simulink model "Fuzzy_Extended_State_Observer_Pendulum"  (R2019a)
settings: Solver=ode1  StartTime=0.0  StopTime=5  FixedStep=0.001  RelTol=1e-3
InitFcn:
  | %Variable_Entrada
  | Phi_max = 200;
  | Phi_2  = 10;
  | Phi_1  = 0.4;
  | Phi_0  = 0;
  | 
  | 
  | %Variable_Salida
  | U_2= 1;
  | U_1 =0.6;
  | U_0  = 0;
  | 
  | 
  | 
  | Phi_max2 = 200;
  | Phi_22  = 10;
  | Phi_12 = 0.3;
  | Phi_02  = 0;
  | 
  | U_22= 1;
  | U_12 =0.7;
  | U_02  = 0;
undefined symbols (not defined in the file or in its folder): fv, g, K, L, l, m
libraries: fuzblock x10, simulink x2
settings Model: Creator=DIEE  LastModifiedBy=dell
settings SolverCC: ZeroCrossAlgorithm=Adaptive
settings DataIOCC: LimitDataPoints=on  SaveFormat=Array  ReturnWorkspaceOutputs=off
settings OptimizationCC: BlockReduction=off  BooleanDataType=off  LifeSpan=inf
settings DebuggingCC: SaveWithParameterizedLinksMsg=none  UnderspecifiedInitializationDetection=Classic  MergeDetectMultiDrivingBlocksExec=none  SignalResolutionControl=TryResolveAllWithWarning  IgnoredZcDiagnostic=none  SFUnexpectedBacktrackingDiag=warning  SFNoUnconditionalDefaultTransitionDiag=warning  SFExecutionAtInitializationDiag=none  ArithmeticOperatorsInVariantConditions=warning
settings HardwareCC: ProdBitPerPointer=32  ProdBitPerSizeT=32  ProdBitPerPtrDiffT=32  ProdLargestAtomicFloat=None  ProdIntDivRoundTo=Undefined  ProdEndianess=Unspecified  ProdWordSize=32  ProdHWDeviceType=32-bit Generic  TargetUnknown=on
settings ModelReferenceCC: PropagateSignalLabelsOutOfModel=off
settings SFSimCC: SimUseLocalCustomCode=off
settings RTWCC: RTWUseLocalCustomCode=off
settings CodeAppCC: StateflowObjectComments=on
settings GRTTargetCC: TargetLangStandard=C89/C90 (ANSI)  GeneratePreprocessorConditionals=Disable all
settings ConfigComp: CovMetricSettings=dw  CovHtmlReporting=on  CovSaveCumulativeToWorkspaceVar=on  CovSaveSingleToWorkspaceVar=on  CovExternalEMLEnable=off  CovSFcnEnable=off

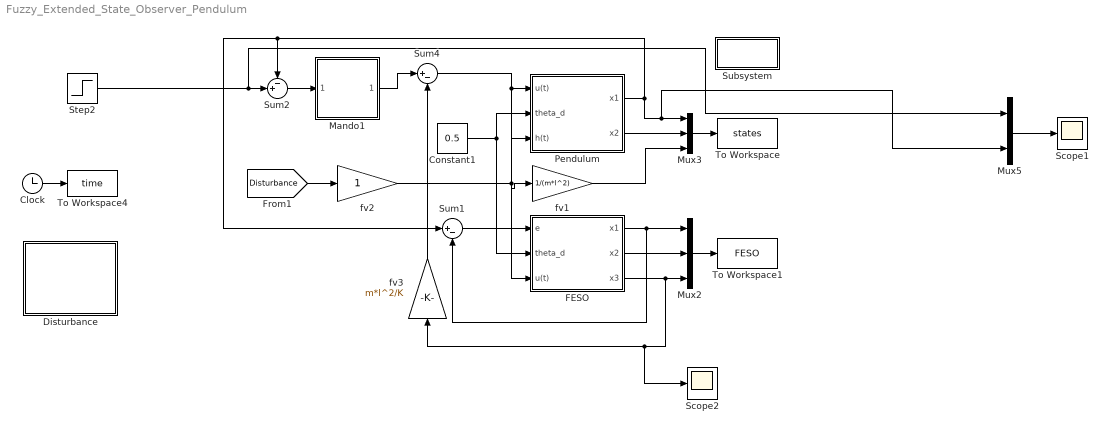
== system Fuzzy_Extended_State_Observer_Pendulum ==
  Clock : Clock
  Constant1 : Constant  Value=0.5
  Disturbance : Subsystem
  FESO : Subsystem
  Mando1 : Subsystem  mask{L=0.1, Kr=0.3, Kp=10, Kd=0.1, Ki=0}
      mask prompts: L "Pendiente"; Kr "Ganancia de Robustez"; Kp "Ganancia proporcional"; Kd "Ganancia derivativa"; Ki "Ganancia Integral"
  Mux2 : Mux  Inputs=3
  Mux3 : Mux  Inputs=3
  Mux5 : Mux  Inputs=2
  Pendulum : Subsystem
  Scope1 : Scope
  Scope2 : Scope
  Step2 : Step  Time=0  After=0.5  SampleTime=0
  Subsystem : Subsystem
      settings: OpenFcn=Plots2
      mask Display: fprintf('PLOT')
  Sum1 : Sum  Inputs=|+-
  Sum2 : Sum  Inputs=-+|
  Sum4 : Sum  Inputs=|+-
  To Workspace : ToWorkspace  VariableName=states  SampleTime=-1
  To Workspace1 : ToWorkspace  VariableName=FESO  SampleTime=-1
  To Workspace4 : ToWorkspace  VariableName=time  SampleTime=-1
  fv1 : Gain  Gain=1/(m*l^2)
  fv2 : Gain
  fv3 : Gain  Gain=m*l^2/K
  wires:
  Pendulum/1(x1) -> Sum1/1, Sum2/1, Mux5/2, Mux3/1
  Mux3/1 -> To Workspace/1
  Pendulum/2(x2) -> Mux3/2
  Constant1/1 -> Pendulum/2(theta_d), FESO/2(theta_d)
  Sum2/1 -> Mando1/1(real_1)
  FESO/2(x2) -> Mux2/2
  FESO/1(x1) -> Sum1/2, Mux2/1
  Mux2/1 -> To Workspace1/1
  Sum1/1 -> FESO/1(e)
  Step2/1 -> Mux5/1, Sum2/2
  Clock/1 -> To Workspace4/1
  Mux5/1 -> Scope1/1
  fv1/1 -> Mux3/3
  [Disturbance] -> fv2/1
  fv2/1 -> fv1/1, Pendulum/3(h(t))
  Mando1/1(mando_1) -> Sum4/1
  Sum4/1 -> FESO/3(u(t)), Pendulum/1(u(t))
  FESO/3(x3) -> Scope2/1, fv3/1, Mux2/3
  fv3/1 -> Sum4/2

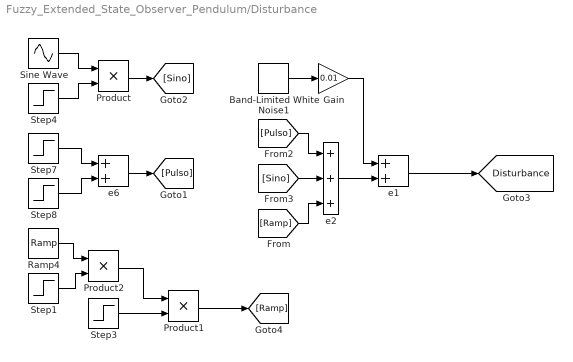
== system Fuzzy_Extended_State_Observer_Pendulum/Disturbance ==
  Band-Limited White Noise1 : simulink/Sources/Band-Limited White Noise  Cov=[0.1]  Ts=0.1  seed=[23341]
  Gain : Gain  Gain=0.01
  Product : Product
  Product1 : Product
  Product2 : Product
  Ramp4 : simulink/Sources/Ramp  slope=1  start=0  InitialOutput=-1
  Sine Wave : Sin  Frequency=2*pi  SampleTime=0
  Step1 : Step  SampleTime=0
  Step3 : Step  Time=2  Before=1  After=0  SampleTime=0
  Step4 : Step  Time=4  SampleTime=0
  Step7 : Step  Time=3  SampleTime=0
  Step8 : Step  Time=4  After=-1  SampleTime=0
  e1 : Sum
  e2 : Sum  Inputs=+++
  e6 : Sum
  tag scope: Disturbance=global
  wires:
  [Sino] -> e2/2
  [Pulso] -> e2/1
  [Ramp] -> e2/3
  Step3/1 -> Product1/2
  Product1/1 -> [Ramp]
  Product2/1 -> Product1/1
  e6/1 -> [Pulso]
  Ramp4/1 -> Product2/1
  Step1/1 -> Product2/2
  Step7/1 -> e6/1
  Step4/1 -> Product/2
  Product/1 -> [Sino]
  Step8/1 -> e6/2
  Sine Wave/1 -> Product/1
  e2/1 -> e1/2
  e1/1 -> [Disturbance]
  Gain/1 -> e1/1
  Band-Limited White Noise1/1 -> Gain/1

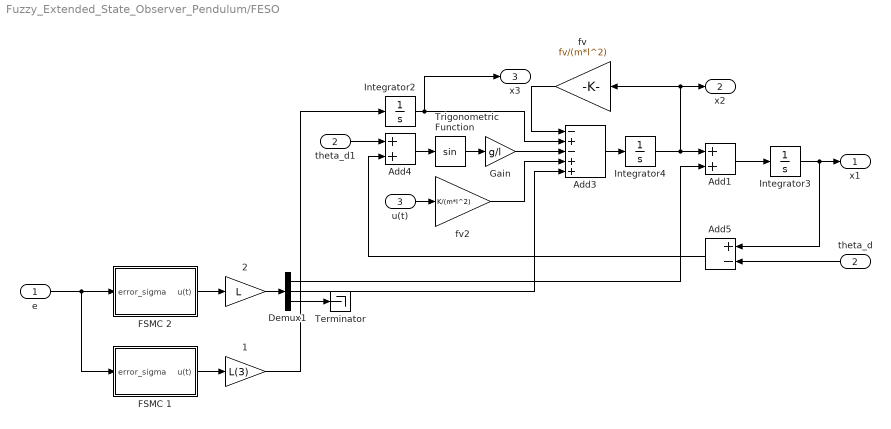
== system Fuzzy_Extended_State_Observer_Pendulum/FESO ==
  e : Inport
  theta_d : Inport  Port=2
  u(t) : Inport  Port=3
  1 : Gain  Gain=L(3)
  2 : Gain  Gain=L
  Add1 : Sum
  Add3 : Sum  Inputs=-+-++
  Add4 : Sum
  Add5 : Sum  Inputs=+-
  Demux1 : Demux  Outputs=3
  FSMC 1 : Subsystem
  FSMC 2 : Subsystem
  Gain : Gain  Gain=g/l
  Integrator2 : Integrator
  Integrator3 : Integrator  InitialCondition=.1
  Integrator4 : Integrator  InitialCondition=0.1
  Terminator : Terminator
  Trigonometric Function : Trigonometry
  fv : Gain  Gain=fv/(m*l^2)
  fv2 : Gain  Gain=K/(m*l^2)
  theta_d1 : InportShadow  Port=2
  x1 : Outport
  x2 : Outport  Port=2
  x3 : Outport  Port=3
  wires:
  fv/1 -> Add3/1
  theta_d1/1 -> Add4/1
  Gain/1 -> Add3/3
  theta_d/1 -> Add5/2
  Add4/1 -> Trigonometric Function/1
  Add5/1 -> Add4/2
  fv2/1 -> Add3/4
  u(t)/1 -> fv2/1
  Integrator3/1 -> Add5/1, x1/1
  Add3/1 -> Integrator4/1
  Trigonometric Function/1 -> Gain/1
  Integrator4/1 -> Add1/1, fv/1, x2/1
  Add1/1 -> Integrator3/1
  Integrator2/1 -> x3/1, Add3/2
  Demux1/2 -> Add3/5
  FSMC 2/1(u(t)) -> 2/1
  FSMC 1/1(u(t)) -> 1/1
  Demux1/1 -> Add1/2
  1/1 -> Integrator2/1
  e/1 -> FSMC 2/1(error_sigma), FSMC 1/1(error_sigma)
  2/1 -> Demux1/1
  Demux1/3 -> Terminator/1

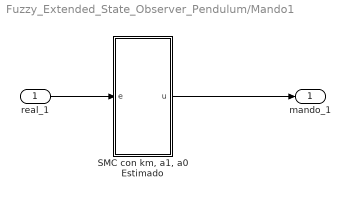
== system Fuzzy_Extended_State_Observer_Pendulum/Mando1 ==
  real_1 : Inport
  "SMC con km, a1, a0 Estimado" : Subsystem  mask{L=L, F=Kr, Kp=Kp, Ki=Ki, Kd=Kd}
      mask prompts: L "Landa(L)"; F "Ganancia robustez(F)"; Kp "Ganancia Proporcional(Kp)"; Ki "Ganancia Integral(Ki)"; Kd "Ganancia derivativa(Kd)"
  mando_1 : Outport
  wires:
  "SMC con km, a1, a0 Estimado"/1(u) -> mando_1/1
  real_1/1 -> "SMC con km, a1, a0 Estimado"/1(e)

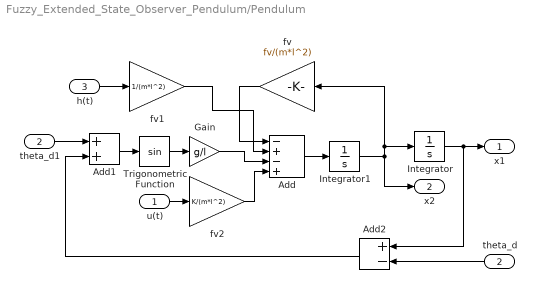
== system Fuzzy_Extended_State_Observer_Pendulum/Pendulum ==
  u(t) : Inport
  theta_d : Inport  Port=2
  h(t) : Inport  Port=3
  Add : Sum  Inputs=-+-+
  Add1 : Sum
  Add2 : Sum  Inputs=+-
  Gain : Gain  Gain=g/l
  Integrator : Integrator  InitialCondition=0.1
  Integrator1 : Integrator  InitialCondition=0.1
  Trigonometric Function : Trigonometry
  fv : Gain  Gain=fv/(m*l^2)
  fv1 : Gain  Gain=1/(m*l^2)
  fv2 : Gain  Gain=K/(m*l^2)
  theta_d1 : InportShadow  Port=2
  x1 : Outport
  x2 : Outport  Port=2
  wires:
  Add/1 -> Integrator1/1
  Integrator1/1 -> fv/1, Integrator/1, x2/1
  fv/1 -> Add/1
  Integrator/1 -> Add2/1, x1/1
  h(t)/1 -> fv1/1
  fv1/1 -> Add/2
  Trigonometric Function/1 -> Gain/1
  Add2/1 -> Add1/2
  u(t)/1 -> fv2/1
  fv2/1 -> Add/4
  Gain/1 -> Add/3
  theta_d/1 -> Add2/2
  Add1/1 -> Trigonometric Function/1
  theta_d1/1 -> Add1/1

== system Fuzzy_Extended_State_Observer_Pendulum/Subsystem ==

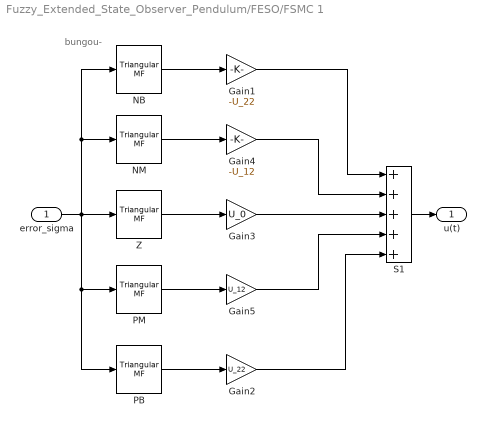
== system Fuzzy_Extended_State_Observer_Pendulum/FESO/FSMC 1 ==
  note: bungou-
  error_sigma : Inport
  Gain1 : Gain  Gain=-U_22
  Gain2 : Gain  Gain=U_22
  Gain3 : Gain  Gain=U_0
  Gain4 : Gain  Gain=-U_12
  Gain5 : Gain  Gain=U_12
  NB : fuzblock/Membership  Functions/Triangular MF  a=-Phi_max  b=-Phi_22  c=-Phi_12
      settings: SourceProductName=Fuzzy Logic Toolbox  SourceProductBaseCode=FL
  NM : fuzblock/Membership  Functions/Triangular MF  a=-Phi_22  b=-Phi_12  c=-Phi_0
      settings: SourceProductName=Fuzzy Logic Toolbox  SourceProductBaseCode=FL
  PB : fuzblock/Membership  Functions/Triangular MF  a=Phi_12  b=Phi_22  c=Phi_max
      settings: SourceProductName=Fuzzy Logic Toolbox  SourceProductBaseCode=FL
  PM : fuzblock/Membership  Functions/Triangular MF  a=Phi_0  b=Phi_12  c=Phi_22
      settings: SourceProductName=Fuzzy Logic Toolbox  SourceProductBaseCode=FL
  S1 : Sum  Inputs=+++++  SaturateOnIntegerOverflow=on  InputSameDT=on  OutDataTypeStr=Inherit: Same as first input
  Z : fuzblock/Membership  Functions/Triangular MF  a=-Phi_12  b=0  c=Phi_12
      settings: SourceProductName=Fuzzy Logic Toolbox  SourceProductBaseCode=FL
  u(t) : Outport
  wires:
  NM/1 -> Gain4/1
  S1/1 -> u(t)/1
  error_sigma/1 -> PM/1, PB/1, Z/1, NM/1, NB/1
  Gain5/1 -> S1/4
  Gain2/1 -> S1/5
  Gain3/1 -> S1/3
  Gain4/1 -> S1/2
  Gain1/1 -> S1/1
  PM/1 -> Gain5/1
  PB/1 -> Gain2/1
  Z/1 -> Gain3/1
  NB/1 -> Gain1/1

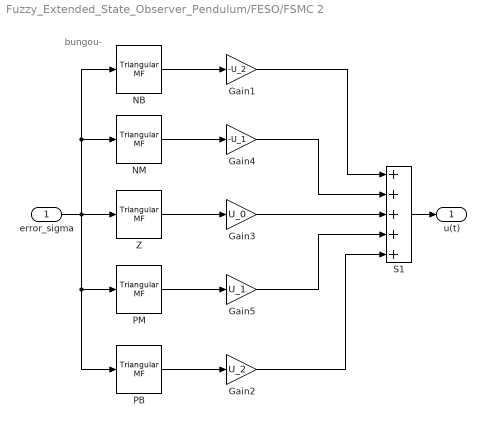
== system Fuzzy_Extended_State_Observer_Pendulum/FESO/FSMC 2 ==
  note: bungou-
  error_sigma : Inport
  Gain1 : Gain  Gain=-U_2
  Gain2 : Gain  Gain=U_2
  Gain3 : Gain  Gain=U_0
  Gain4 : Gain  Gain=-U_1
  Gain5 : Gain  Gain=U_1
  NB : fuzblock/Membership  Functions/Triangular MF  a=-Phi_max  b=-Phi_2  c=-Phi_1
      settings: SourceProductName=Fuzzy Logic Toolbox  SourceProductBaseCode=FL
  NM : fuzblock/Membership  Functions/Triangular MF  a=-Phi_2  b=-Phi_1  c=-Phi_0
      settings: SourceProductName=Fuzzy Logic Toolbox  SourceProductBaseCode=FL
  PB : fuzblock/Membership  Functions/Triangular MF  a=Phi_1  b=Phi_2  c=Phi_max
      settings: SourceProductName=Fuzzy Logic Toolbox  SourceProductBaseCode=FL
  PM : fuzblock/Membership  Functions/Triangular MF  a=Phi_0  b=Phi_1  c=Phi_2
      settings: SourceProductName=Fuzzy Logic Toolbox  SourceProductBaseCode=FL
  S1 : Sum  Inputs=+++++  SaturateOnIntegerOverflow=on  InputSameDT=on  OutDataTypeStr=Inherit: Same as first input
  Z : fuzblock/Membership  Functions/Triangular MF  a=-Phi_1  b=0  c=Phi_1
      settings: SourceProductName=Fuzzy Logic Toolbox  SourceProductBaseCode=FL
  u(t) : Outport
  wires:
  NM/1 -> Gain4/1
  S1/1 -> u(t)/1
  error_sigma/1 -> PM/1, PB/1, Z/1, NM/1, NB/1
  Gain5/1 -> S1/4
  Gain2/1 -> S1/5
  Gain3/1 -> S1/3
  Gain4/1 -> S1/2
  Gain1/1 -> S1/1
  PM/1 -> Gain5/1
  PB/1 -> Gain2/1
  Z/1 -> Gain3/1
  NB/1 -> Gain1/1

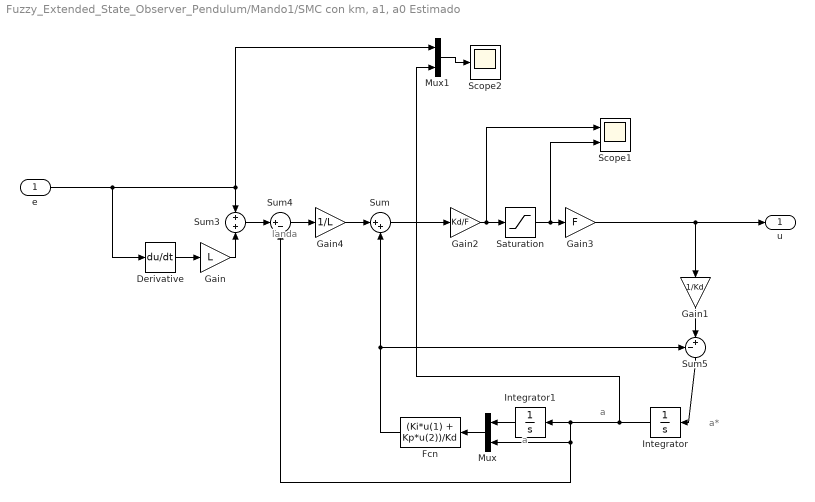
== system Fuzzy_Extended_State_Observer_Pendulum/Mando1/SMC con km, a1, a0 Estimado ==
  note: a
  note: a
  note: a*
  note: landa
  e : Inport
  Derivative : Derivative
  Fcn : Fcn  Expr=(Ki*u(1) + Kp*u(2))/Kd
  Gain : Gain  Gain=L
  Gain1 : Gain  Gain=1/Kd
  Gain2 : Gain  Gain=Kd/F
  Gain3 : Gain  Gain=F
  Gain4 : Gain  Gain=1/L
  Integrator : Integrator  UpperSaturationLimit=5  LowerSaturationLimit=-5
  Integrator1 : Integrator  UpperSaturationLimit=1  LowerSaturationLimit=-1
  Mux : Mux  Inputs=2
  Mux1 : Mux  Inputs=2
  Saturation : Saturate  UpperLimit=1  LowerLimit=-1
  Scope1 : Scope  NumInputPorts=2
  Scope2 : Scope
  Sum : Sum  Inputs=|++
  Sum3 : Sum  Inputs=+|+
  Sum4 : Sum  Inputs=|+-
  Sum5 : Sum  Inputs=-+|
  u : Outport
  wires:
  Mux1/1 -> Scope2/1
  e/1 -> Derivative/1, Sum3/1, Mux1/1
  Integrator1/1 -> Mux/1
  Gain3/1 -> u/1, Gain1/1
  Gain4/1 -> Sum/1
  Sum4/1 -> Gain4/1
  Mux/1 -> Fcn/1
  Integrator/1 -> Sum4/2, Mux/2, Integrator1/1, Mux1/2
  Sum5/1 -> Integrator/1
  Fcn/1 -> Sum5/1, Sum/2
  Gain1/1 -> Sum5/2
  Saturation/1 -> Gain3/1, Scope1/2
  Sum/1 -> Gain2/1
  Gain2/1 -> Saturation/1, Scope1/1
  Sum3/1 -> Sum4/1
  Gain/1 -> Sum3/2
  Derivative/1 -> Gain/1
